simulink model "Block Diagram"  (R2024b)
settings: Solver=VariableStepAuto  StartTime=0.0  StopTime=10.0  RelTol=1e-3
libraries: simulink_extras x43, eeGeneralControl x4
(part 2 of 3)

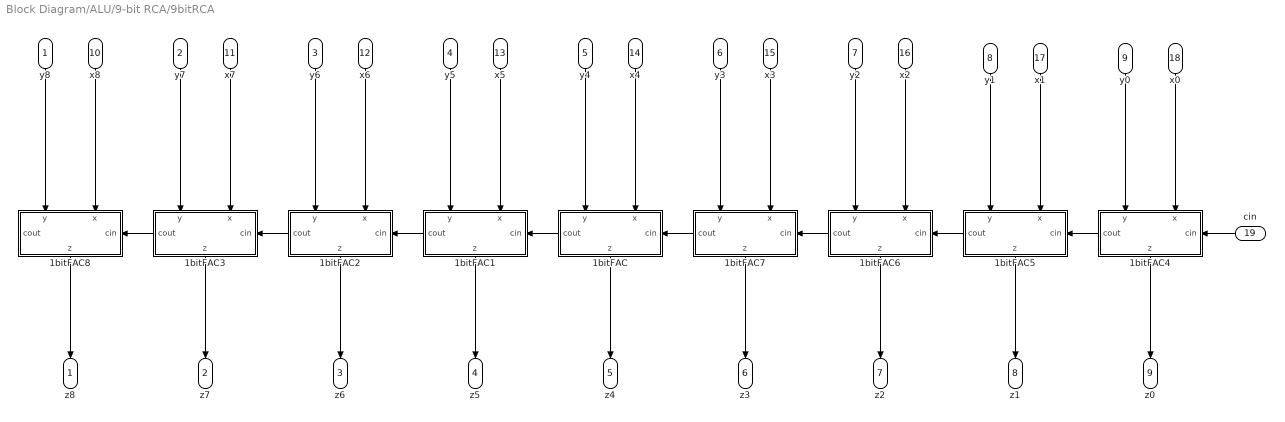
== system Block Diagram/ALU/9-bit RCA/9bitRCA ==
  y8 : Inport
  y7 : Inport  Port=2
  y6 : Inport  Port=3
  y5 : Inport  Port=4
  y4 : Inport  Port=5
  y3 : Inport  Port=6
  y2 : Inport  Port=7
  y1 : Inport  Port=8
  y0 : Inport  Port=9
  x8 : Inport  Port=10
  x7 : Inport  Port=11
  x6 : Inport  Port=12
  x5 : Inport  Port=13
  x4 : Inport  Port=14
  x3 : Inport  Port=15
  x2 : Inport  Port=16
  x1 : Inport  Port=17
  x0 : Inport  Port=18
  cin : Inport  Port=19
  1bitFAC : Subsystem
      settings: PortSchema="{\"entries\":[{\"content\":{\"sides\":[{\"content\":{\"connectorIds\":[\"Out2\"]},\"type\":\"ConnectorPlacement.EquallySpacedRectSide\",\"uuid\":\"3d82b7f9-dc63-4fc7-98b7-23cc47f57a4f\"},{\"content\":{\"connectorIds\":[\"In3\"],\"side\":\"RIGHT\"},\"type\":\"ConnectorPlacement.EquallySpacedRectSide\",\"uuid\":\"46fdb482-606a-4080-9fe4-28ef2e2aeced\"},{\"content\":{\"connectorIds\":[\"In1\",\"In2\"],\"side\":\"TOP\"},\"type\":\"ConnectorPlacement.EquallySpacedRectSide\",\"uuid\":\"27deceb1-bcd8-433c-80a1-5ff3de271941\"},{\"content\":{\"connectorIds\":[\"Out1\"],\"side\":\"BOTTOM\"},\"type\":\"ConnectorPlacement.EquallySpacedRectSide\",\"uuid\":\"1ab1ef58-b8ab-498e-bc4b-e7d01d078e9d\"}]},\"type\":\"ConnectorPlacement.EquallySpacedConnector\",\"uuid\":\"ca739cf1-46eb-41bd-970c-7d220730d652\"}],\"packageUris\":[\"http://schema.mathworks.com/mf0/Connector/R2020b\"],\"version\":\"1.0\"}"
  1bitFAC1 : Subsystem
      settings: PortSchema="{\"entries\":[{\"content\":{\"sides\":[{\"content\":{\"connectorIds\":[\"Out2\"]},\"type\":\"ConnectorPlacement.EquallySpacedRectSide\",\"uuid\":\"3d82b7f9-dc63-4fc7-98b7-23cc47f57a4f\"},{\"content\":{\"connectorIds\":[\"In3\"],\"side\":\"RIGHT\"},\"type\":\"ConnectorPlacement.EquallySpacedRectSide\",\"uuid\":\"46fdb482-606a-4080-9fe4-28ef2e2aeced\"},{\"content\":{\"connectorIds\":[\"In1\",\"In2\"],\"side\":\"TOP\"},\"type\":\"ConnectorPlacement.EquallySpacedRectSide\",\"uuid\":\"27deceb1-bcd8-433c-80a1-5ff3de271941\"},{\"content\":{\"connectorIds\":[\"Out1\"],\"side\":\"BOTTOM\"},\"type\":\"ConnectorPlacement.EquallySpacedRectSide\",\"uuid\":\"1ab1ef58-b8ab-498e-bc4b-e7d01d078e9d\"}]},\"type\":\"ConnectorPlacement.EquallySpacedConnector\",\"uuid\":\"ca739cf1-46eb-41bd-970c-7d220730d652\"}],\"packageUris\":[\"http://schema.mathworks.com/mf0/Connector/R2020b\"],\"version\":\"1.0\"}"
  1bitFAC2 : Subsystem
      settings: PortSchema="{\"entries\":[{\"content\":{\"sides\":[{\"content\":{\"connectorIds\":[\"Out2\"]},\"type\":\"ConnectorPlacement.EquallySpacedRectSide\",\"uuid\":\"3d82b7f9-dc63-4fc7-98b7-23cc47f57a4f\"},{\"content\":{\"connectorIds\":[\"In3\"],\"side\":\"RIGHT\"},\"type\":\"ConnectorPlacement.EquallySpacedRectSide\",\"uuid\":\"46fdb482-606a-4080-9fe4-28ef2e2aeced\"},{\"content\":{\"connectorIds\":[\"In1\",\"In2\"],\"side\":\"TOP\"},\"type\":\"ConnectorPlacement.EquallySpacedRectSide\",\"uuid\":\"27deceb1-bcd8-433c-80a1-5ff3de271941\"},{\"content\":{\"connectorIds\":[\"Out1\"],\"side\":\"BOTTOM\"},\"type\":\"ConnectorPlacement.EquallySpacedRectSide\",\"uuid\":\"1ab1ef58-b8ab-498e-bc4b-e7d01d078e9d\"}]},\"type\":\"ConnectorPlacement.EquallySpacedConnector\",\"uuid\":\"ca739cf1-46eb-41bd-970c-7d220730d652\"}],\"packageUris\":[\"http://schema.mathworks.com/mf0/Connector/R2020b\"],\"version\":\"1.0\"}"
  1bitFAC3 : Subsystem
      settings: PortSchema="{\"entries\":[{\"content\":{\"sides\":[{\"content\":{\"connectorIds\":[\"Out2\"]},\"type\":\"ConnectorPlacement.EquallySpacedRectSide\",\"uuid\":\"3d82b7f9-dc63-4fc7-98b7-23cc47f57a4f\"},{\"content\":{\"connectorIds\":[\"In3\"],\"side\":\"RIGHT\"},\"type\":\"ConnectorPlacement.EquallySpacedRectSide\",\"uuid\":\"46fdb482-606a-4080-9fe4-28ef2e2aeced\"},{\"content\":{\"connectorIds\":[\"In1\",\"In2\"],\"side\":\"TOP\"},\"type\":\"ConnectorPlacement.EquallySpacedRectSide\",\"uuid\":\"27deceb1-bcd8-433c-80a1-5ff3de271941\"},{\"content\":{\"connectorIds\":[\"Out1\"],\"side\":\"BOTTOM\"},\"type\":\"ConnectorPlacement.EquallySpacedRectSide\",\"uuid\":\"1ab1ef58-b8ab-498e-bc4b-e7d01d078e9d\"}]},\"type\":\"ConnectorPlacement.EquallySpacedConnector\",\"uuid\":\"ca739cf1-46eb-41bd-970c-7d220730d652\"}],\"packageUris\":[\"http://schema.mathworks.com/mf0/Connector/R2020b\"],\"version\":\"1.0\"}"
  1bitFAC4 : Subsystem
      settings: PortSchema="{\"entries\":[{\"content\":{\"sides\":[{\"content\":{\"connectorIds\":[\"Out2\"]},\"type\":\"ConnectorPlacement.EquallySpacedRectSide\",\"uuid\":\"3d82b7f9-dc63-4fc7-98b7-23cc47f57a4f\"},{\"content\":{\"connectorIds\":[\"In3\"],\"side\":\"RIGHT\"},\"type\":\"ConnectorPlacement.EquallySpacedRectSide\",\"uuid\":\"46fdb482-606a-4080-9fe4-28ef2e2aeced\"},{\"content\":{\"connectorIds\":[\"In1\",\"In2\"],\"side\":\"TOP\"},\"type\":\"ConnectorPlacement.EquallySpacedRectSide\",\"uuid\":\"27deceb1-bcd8-433c-80a1-5ff3de271941\"},{\"content\":{\"connectorIds\":[\"Out1\"],\"side\":\"BOTTOM\"},\"type\":\"ConnectorPlacement.EquallySpacedRectSide\",\"uuid\":\"1ab1ef58-b8ab-498e-bc4b-e7d01d078e9d\"}]},\"type\":\"ConnectorPlacement.EquallySpacedConnector\",\"uuid\":\"ca739cf1-46eb-41bd-970c-7d220730d652\"}],\"packageUris\":[\"http://schema.mathworks.com/mf0/Connector/R2020b\"],\"version\":\"1.0\"}"
  1bitFAC5 : Subsystem
      settings: PortSchema="{\"entries\":[{\"content\":{\"sides\":[{\"content\":{\"connectorIds\":[\"Out2\"]},\"type\":\"ConnectorPlacement.EquallySpacedRectSide\",\"uuid\":\"3d82b7f9-dc63-4fc7-98b7-23cc47f57a4f\"},{\"content\":{\"connectorIds\":[\"In3\"],\"side\":\"RIGHT\"},\"type\":\"ConnectorPlacement.EquallySpacedRectSide\",\"uuid\":\"46fdb482-606a-4080-9fe4-28ef2e2aeced\"},{\"content\":{\"connectorIds\":[\"In1\",\"In2\"],\"side\":\"TOP\"},\"type\":\"ConnectorPlacement.EquallySpacedRectSide\",\"uuid\":\"27deceb1-bcd8-433c-80a1-5ff3de271941\"},{\"content\":{\"connectorIds\":[\"Out1\"],\"side\":\"BOTTOM\"},\"type\":\"ConnectorPlacement.EquallySpacedRectSide\",\"uuid\":\"1ab1ef58-b8ab-498e-bc4b-e7d01d078e9d\"}]},\"type\":\"ConnectorPlacement.EquallySpacedConnector\",\"uuid\":\"ca739cf1-46eb-41bd-970c-7d220730d652\"}],\"packageUris\":[\"http://schema.mathworks.com/mf0/Connector/R2020b\"],\"version\":\"1.0\"}"
  1bitFAC6 : Subsystem
      settings: PortSchema="{\"entries\":[{\"content\":{\"sides\":[{\"content\":{\"connectorIds\":[\"Out2\"]},\"type\":\"ConnectorPlacement.EquallySpacedRectSide\",\"uuid\":\"3d82b7f9-dc63-4fc7-98b7-23cc47f57a4f\"},{\"content\":{\"connectorIds\":[\"In3\"],\"side\":\"RIGHT\"},\"type\":\"ConnectorPlacement.EquallySpacedRectSide\",\"uuid\":\"46fdb482-606a-4080-9fe4-28ef2e2aeced\"},{\"content\":{\"connectorIds\":[\"In1\",\"In2\"],\"side\":\"TOP\"},\"type\":\"ConnectorPlacement.EquallySpacedRectSide\",\"uuid\":\"27deceb1-bcd8-433c-80a1-5ff3de271941\"},{\"content\":{\"connectorIds\":[\"Out1\"],\"side\":\"BOTTOM\"},\"type\":\"ConnectorPlacement.EquallySpacedRectSide\",\"uuid\":\"1ab1ef58-b8ab-498e-bc4b-e7d01d078e9d\"}]},\"type\":\"ConnectorPlacement.EquallySpacedConnector\",\"uuid\":\"ca739cf1-46eb-41bd-970c-7d220730d652\"}],\"packageUris\":[\"http://schema.mathworks.com/mf0/Connector/R2020b\"],\"version\":\"1.0\"}"
  1bitFAC7 : Subsystem
      settings: PortSchema="{\"entries\":[{\"content\":{\"sides\":[{\"content\":{\"connectorIds\":[\"Out2\"]},\"type\":\"ConnectorPlacement.EquallySpacedRectSide\",\"uuid\":\"3d82b7f9-dc63-4fc7-98b7-23cc47f57a4f\"},{\"content\":{\"connectorIds\":[\"In3\"],\"side\":\"RIGHT\"},\"type\":\"ConnectorPlacement.EquallySpacedRectSide\",\"uuid\":\"46fdb482-606a-4080-9fe4-28ef2e2aeced\"},{\"content\":{\"connectorIds\":[\"In1\",\"In2\"],\"side\":\"TOP\"},\"type\":\"ConnectorPlacement.EquallySpacedRectSide\",\"uuid\":\"27deceb1-bcd8-433c-80a1-5ff3de271941\"},{\"content\":{\"connectorIds\":[\"Out1\"],\"side\":\"BOTTOM\"},\"type\":\"ConnectorPlacement.EquallySpacedRectSide\",\"uuid\":\"1ab1ef58-b8ab-498e-bc4b-e7d01d078e9d\"}]},\"type\":\"ConnectorPlacement.EquallySpacedConnector\",\"uuid\":\"ca739cf1-46eb-41bd-970c-7d220730d652\"}],\"packageUris\":[\"http://schema.mathworks.com/mf0/Connector/R2020b\"],\"version\":\"1.0\"}"
  1bitFAC8 : Subsystem
      settings: PortSchema="{\"entries\":[{\"content\":{\"sides\":[{\"content\":{\"connectorIds\":[\"Out2\"]},\"type\":\"ConnectorPlacement.EquallySpacedRectSide\",\"uuid\":\"3d82b7f9-dc63-4fc7-98b7-23cc47f57a4f\"},{\"content\":{\"connectorIds\":[\"In3\"],\"side\":\"RIGHT\"},\"type\":\"ConnectorPlacement.EquallySpacedRectSide\",\"uuid\":\"46fdb482-606a-4080-9fe4-28ef2e2aeced\"},{\"content\":{\"connectorIds\":[\"In1\",\"In2\"],\"side\":\"TOP\"},\"type\":\"ConnectorPlacement.EquallySpacedRectSide\",\"uuid\":\"27deceb1-bcd8-433c-80a1-5ff3de271941\"},{\"content\":{\"connectorIds\":[\"Out1\"],\"side\":\"BOTTOM\"},\"type\":\"ConnectorPlacement.EquallySpacedRectSide\",\"uuid\":\"1ab1ef58-b8ab-498e-bc4b-e7d01d078e9d\"}]},\"type\":\"ConnectorPlacement.EquallySpacedConnector\",\"uuid\":\"ca739cf1-46eb-41bd-970c-7d220730d652\"}],\"packageUris\":[\"http://schema.mathworks.com/mf0/Connector/R2020b\"],\"version\":\"1.0\"}"
  z8 : Outport
  z7 : Outport  Port=2
  z6 : Outport  Port=3
  z5 : Outport  Port=4
  z4 : Outport  Port=5
  z3 : Outport  Port=6
  z2 : Outport  Port=7
  z1 : Outport  Port=8
  z0 : Outport  Port=9
  wires:
  1bitFAC1/2(cout) -> 1bitFAC2/3(cin)
  1bitFAC5/2(cout) -> 1bitFAC6/3(cin)
  1bitFAC3/2(cout) -> 1bitFAC8/3(cin)
  1bitFAC2/2(cout) -> 1bitFAC3/3(cin)
  1bitFAC/2(cout) -> 1bitFAC1/3(cin)
  1bitFAC7/2(cout) -> 1bitFAC/3(cin)
  1bitFAC6/2(cout) -> 1bitFAC7/3(cin)
  1bitFAC4/2(cout) -> 1bitFAC5/3(cin)
  x0/1 -> 1bitFAC4/2(x)
  x1/1 -> 1bitFAC5/2(x)
  x2/1 -> 1bitFAC6/2(x)
  x3/1 -> 1bitFAC7/2(x)
  x4/1 -> 1bitFAC/2(x)
  x5/1 -> 1bitFAC1/2(x)
  x6/1 -> 1bitFAC2/2(x)
  x7/1 -> 1bitFAC3/2(x)
  x8/1 -> 1bitFAC8/2(x)
  y5/1 -> 1bitFAC1/1(y)
  y7/1 -> 1bitFAC3/1(y)
  y6/1 -> 1bitFAC2/1(y)
  y1/1 -> 1bitFAC5/1(y)
  y4/1 -> 1bitFAC/1(y)
  y2/1 -> 1bitFAC6/1(y)
  y0/1 -> 1bitFAC4/1(y)
  y8/1 -> 1bitFAC8/1(y)
  y3/1 -> 1bitFAC7/1(y)
  1bitFAC4/1(z) -> z0/1
  1bitFAC5/1(z) -> z1/1
  1bitFAC6/1(z) -> z2/1
  1bitFAC7/1(z) -> z3/1
  1bitFAC/1(z) -> z4/1
  1bitFAC1/1(z) -> z5/1
  1bitFAC2/1(z) -> z6/1
  1bitFAC3/1(z) -> z7/1
  1bitFAC8/1(z) -> z8/1
  cin/1 -> 1bitFAC4/3(cin)

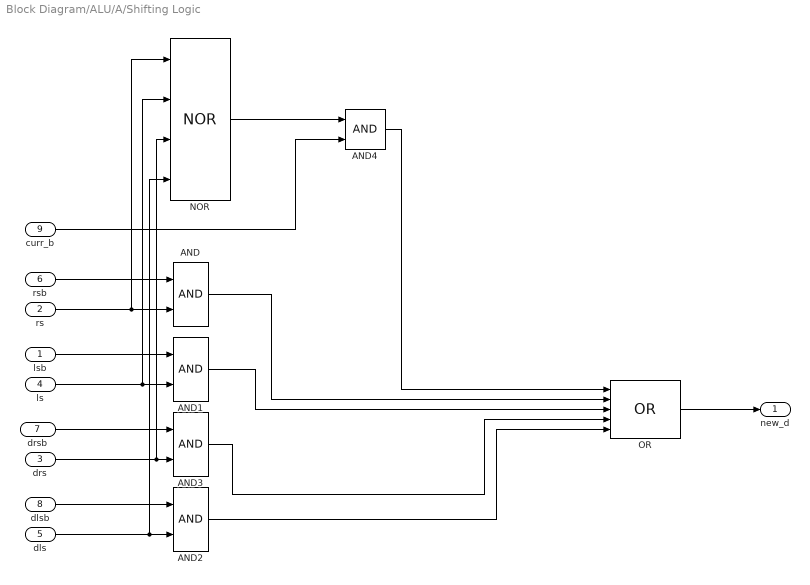
== system Block Diagram/ALU/A/Shifting Logic ==
  lsb : Inport
  rs : Inport  Port=2
  drs : Inport  Port=3
  ls : Inport  Port=4
  dls : Inport  Port=5
  rsb : Inport  Port=6
  drsb : Inport  Port=7
  dlsb : Inport  Port=8
  curr_b : Inport  Port=9
  AND{,1..4} (5 alike) : Logic  IconShape=distinctive  AllPortsSameDT=off  OutDataTypeStr=boolean
  NOR : Logic  Operator=NOR  Inputs=4  IconShape=distinctive  AllPortsSameDT=off  OutDataTypeStr=boolean
  OR : Logic  Operator=OR  Inputs=5  IconShape=distinctive  AllPortsSameDT=off  OutDataTypeStr=boolean
  new_d : Outport
  wires:
  curr_b/1 -> AND4/2
  rsb/1 -> AND/1
  rs/1 -> NOR/1, AND/2
  lsb/1 -> AND1/1
  ls/1 -> NOR/2, AND1/2
  drs/1 -> NOR/3, AND3/2
  drsb/1 -> AND3/1
  dls/1 -> NOR/4, AND2/2
  dlsb/1 -> AND2/1
  NOR/1 -> AND4/1
  AND/1 -> OR/2
  AND1/1 -> OR/3
  AND3/1 -> OR/4
  AND2/1 -> OR/5
  AND4/1 -> OR/1
  OR/1 -> new_d/1

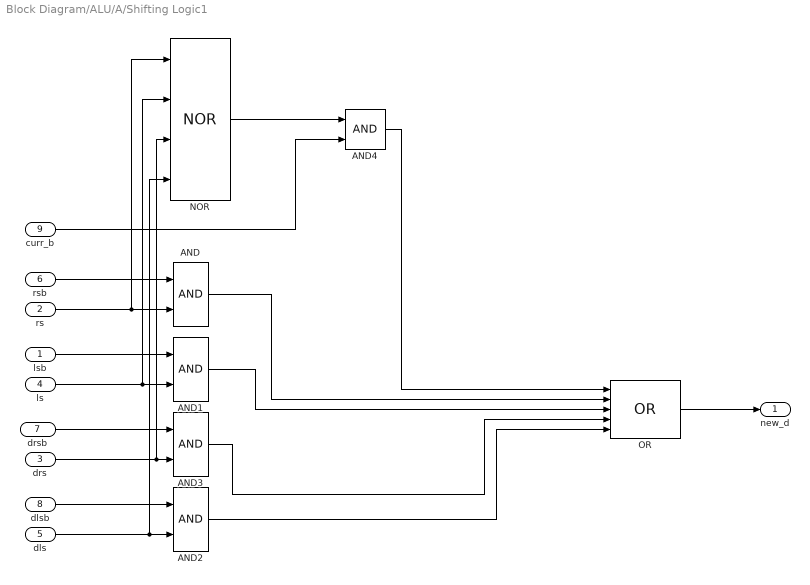
== system Block Diagram/ALU/A/Shifting Logic1 ==
  lsb : Inport
  rs : Inport  Port=2
  drs : Inport  Port=3
  ls : Inport  Port=4
  dls : Inport  Port=5
  rsb : Inport  Port=6
  drsb : Inport  Port=7
  dlsb : Inport  Port=8
  curr_b : Inport  Port=9
  AND{,1..4} (5 alike) : Logic  IconShape=distinctive  AllPortsSameDT=off  OutDataTypeStr=boolean
  NOR : Logic  Operator=NOR  Inputs=4  IconShape=distinctive  AllPortsSameDT=off  OutDataTypeStr=boolean
  OR : Logic  Operator=OR  Inputs=5  IconShape=distinctive  AllPortsSameDT=off  OutDataTypeStr=boolean
  new_d : Outport
  wires:
  curr_b/1 -> AND4/2
  rsb/1 -> AND/1
  rs/1 -> NOR/1, AND/2
  lsb/1 -> AND1/1
  ls/1 -> NOR/2, AND1/2
  drs/1 -> NOR/3, AND3/2
  drsb/1 -> AND3/1
  dls/1 -> NOR/4, AND2/2
  dlsb/1 -> AND2/1
  NOR/1 -> AND4/1
  AND/1 -> OR/2
  AND1/1 -> OR/3
  AND3/1 -> OR/4
  AND2/1 -> OR/5
  AND4/1 -> OR/1
  OR/1 -> new_d/1

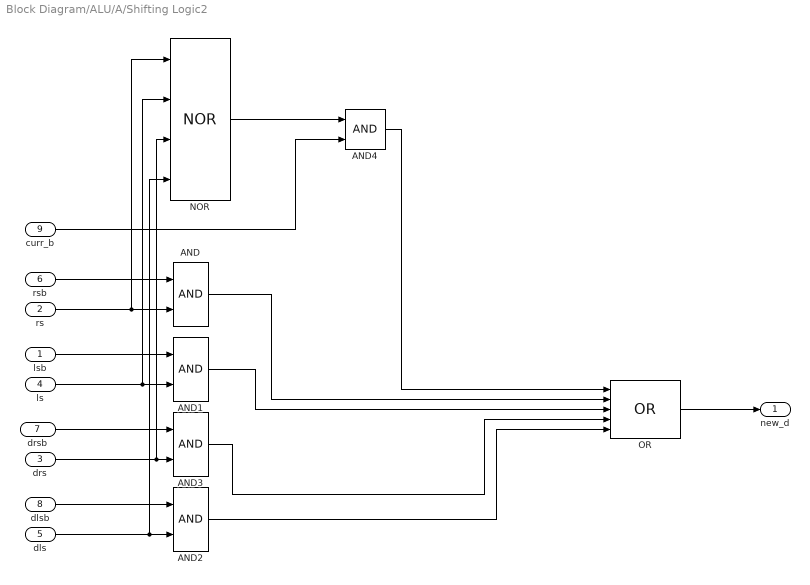
== system Block Diagram/ALU/A/Shifting Logic2 ==
  lsb : Inport
  rs : Inport  Port=2
  drs : Inport  Port=3
  ls : Inport  Port=4
  dls : Inport  Port=5
  rsb : Inport  Port=6
  drsb : Inport  Port=7
  dlsb : Inport  Port=8
  curr_b : Inport  Port=9
  AND{,1..4} (5 alike) : Logic  IconShape=distinctive  AllPortsSameDT=off  OutDataTypeStr=boolean
  NOR : Logic  Operator=NOR  Inputs=4  IconShape=distinctive  AllPortsSameDT=off  OutDataTypeStr=boolean
  OR : Logic  Operator=OR  Inputs=5  IconShape=distinctive  AllPortsSameDT=off  OutDataTypeStr=boolean
  new_d : Outport
  wires:
  curr_b/1 -> AND4/2
  rsb/1 -> AND/1
  rs/1 -> NOR/1, AND/2
  lsb/1 -> AND1/1
  ls/1 -> NOR/2, AND1/2
  drs/1 -> NOR/3, AND3/2
  drsb/1 -> AND3/1
  dls/1 -> NOR/4, AND2/2
  dlsb/1 -> AND2/1
  NOR/1 -> AND4/1
  AND/1 -> OR/2
  AND1/1 -> OR/3
  AND3/1 -> OR/4
  AND2/1 -> OR/5
  AND4/1 -> OR/1
  OR/1 -> new_d/1

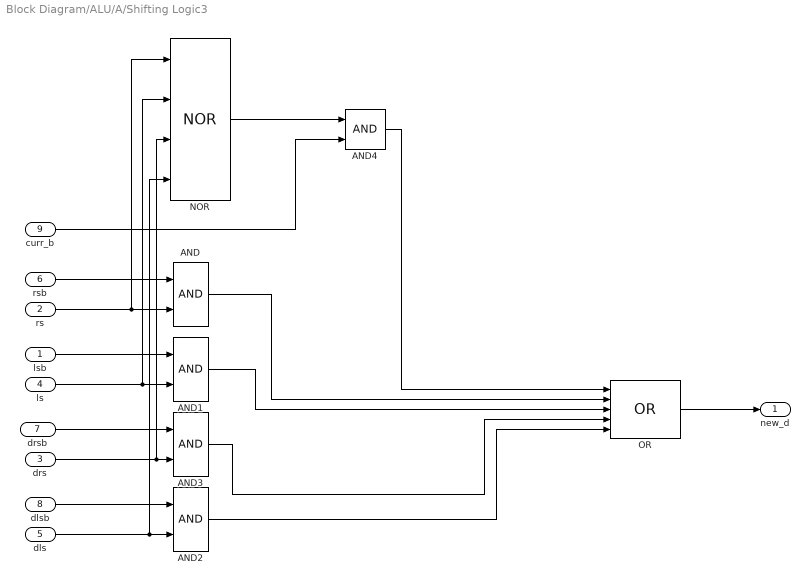
== system Block Diagram/ALU/A/Shifting Logic3 ==
  lsb : Inport
  rs : Inport  Port=2
  drs : Inport  Port=3
  ls : Inport  Port=4
  dls : Inport  Port=5
  rsb : Inport  Port=6
  drsb : Inport  Port=7
  dlsb : Inport  Port=8
  curr_b : Inport  Port=9
  AND{,1..4} (5 alike) : Logic  IconShape=distinctive  AllPortsSameDT=off  OutDataTypeStr=boolean
  NOR : Logic  Operator=NOR  Inputs=4  IconShape=distinctive  AllPortsSameDT=off  OutDataTypeStr=boolean
  OR : Logic  Operator=OR  Inputs=5  IconShape=distinctive  AllPortsSameDT=off  OutDataTypeStr=boolean
  new_d : Outport
  wires:
  curr_b/1 -> AND4/2
  rsb/1 -> AND/1
  rs/1 -> NOR/1, AND/2
  lsb/1 -> AND1/1
  ls/1 -> NOR/2, AND1/2
  drs/1 -> NOR/3, AND3/2
  drsb/1 -> AND3/1
  dls/1 -> NOR/4, AND2/2
  dlsb/1 -> AND2/1
  NOR/1 -> AND4/1
  AND/1 -> OR/2
  AND1/1 -> OR/3
  AND3/1 -> OR/4
  AND2/1 -> OR/5
  AND4/1 -> OR/1
  OR/1 -> new_d/1

== system Block Diagram/ALU/A/Shifting Logic4 ==
  lsb : Inport
  rs : Inport  Port=2
  drs : Inport  Port=3
  ls : Inport  Port=4
  dls : Inport  Port=5
  rsb : Inport  Port=6
  drsb : Inport  Port=7
  dlsb : Inport  Port=8
  curr_b : Inport  Port=9
  AND{,1..4} (5 alike) : Logic  IconShape=distinctive  AllPortsSameDT=off  OutDataTypeStr=boolean
  NOR : Logic  Operator=NOR  Inputs=4  IconShape=distinctive  AllPortsSameDT=off  OutDataTypeStr=boolean
  OR : Logic  Operator=OR  Inputs=5  IconShape=distinctive  AllPortsSameDT=off  OutDataTypeStr=boolean
  new_d : Outport
  wires:
  curr_b/1 -> AND4/2
  rsb/1 -> AND/1
  rs/1 -> NOR/1, AND/2
  lsb/1 -> AND1/1
  ls/1 -> NOR/2, AND1/2
  drs/1 -> NOR/3, AND3/2
  drsb/1 -> AND3/1
  dls/1 -> NOR/4, AND2/2
  dlsb/1 -> AND2/1
  NOR/1 -> AND4/1
  AND/1 -> OR/2
  AND1/1 -> OR/3
  AND3/1 -> OR/4
  AND2/1 -> OR/5
  AND4/1 -> OR/1
  OR/1 -> new_d/1

== system Block Diagram/ALU/A/Shifting Logic5 ==
  lsb : Inport
  rs : Inport  Port=2
  drs : Inport  Port=3
  ls : Inport  Port=4
  dls : Inport  Port=5
  rsb : Inport  Port=6
  drsb : Inport  Port=7
  dlsb : Inport  Port=8
  curr_b : Inport  Port=9
  AND{,1..4} (5 alike) : Logic  IconShape=distinctive  AllPortsSameDT=off  OutDataTypeStr=boolean
  NOR : Logic  Operator=NOR  Inputs=4  IconShape=distinctive  AllPortsSameDT=off  OutDataTypeStr=boolean
  OR : Logic  Operator=OR  Inputs=5  IconShape=distinctive  AllPortsSameDT=off  OutDataTypeStr=boolean
  new_d : Outport
  wires:
  curr_b/1 -> AND4/2
  rsb/1 -> AND/1
  rs/1 -> NOR/1, AND/2
  lsb/1 -> AND1/1
  ls/1 -> NOR/2, AND1/2
  drs/1 -> NOR/3, AND3/2
  drsb/1 -> AND3/1
  dls/1 -> NOR/4, AND2/2
  dlsb/1 -> AND2/1
  NOR/1 -> AND4/1
  AND/1 -> OR/2
  AND1/1 -> OR/3
  AND3/1 -> OR/4
  AND2/1 -> OR/5
  AND4/1 -> OR/1
  OR/1 -> new_d/1

== system Block Diagram/ALU/A/Shifting Logic6 ==
  lsb : Inport
  rs : Inport  Port=2
  drs : Inport  Port=3
  ls : Inport  Port=4
  dls : Inport  Port=5
  rsb : Inport  Port=6
  drsb : Inport  Port=7
  dlsb : Inport  Port=8
  curr_b : Inport  Port=9
  AND{,1..4} (5 alike) : Logic  IconShape=distinctive  AllPortsSameDT=off  OutDataTypeStr=boolean
  NOR : Logic  Operator=NOR  Inputs=4  IconShape=distinctive  AllPortsSameDT=off  OutDataTypeStr=boolean
  OR : Logic  Operator=OR  Inputs=5  IconShape=distinctive  AllPortsSameDT=off  OutDataTypeStr=boolean
  new_d : Outport
  wires:
  curr_b/1 -> AND4/2
  rsb/1 -> AND/1
  rs/1 -> NOR/1, AND/2
  lsb/1 -> AND1/1
  ls/1 -> NOR/2, AND1/2
  drs/1 -> NOR/3, AND3/2
  drsb/1 -> AND3/1
  dls/1 -> NOR/4, AND2/2
  dlsb/1 -> AND2/1
  NOR/1 -> AND4/1
  AND/1 -> OR/2
  AND1/1 -> OR/3
  AND3/1 -> OR/4
  AND2/1 -> OR/5
  AND4/1 -> OR/1
  OR/1 -> new_d/1

== system Block Diagram/ALU/A/Shifting Logic7 ==
  lsb : Inport
  rs : Inport  Port=2
  drs : Inport  Port=3
  ls : Inport  Port=4
  dls : Inport  Port=5
  rsb : Inport  Port=6
  drsb : Inport  Port=7
  dlsb : Inport  Port=8
  curr_b : Inport  Port=9
  AND{,1..4} (5 alike) : Logic  IconShape=distinctive  AllPortsSameDT=off  OutDataTypeStr=boolean
  NOR : Logic  Operator=NOR  Inputs=4  IconShape=distinctive  AllPortsSameDT=off  OutDataTypeStr=boolean
  OR : Logic  Operator=OR  Inputs=5  IconShape=distinctive  AllPortsSameDT=off  OutDataTypeStr=boolean
  new_d : Outport
  wires:
  curr_b/1 -> AND4/2
  rsb/1 -> AND/1
  rs/1 -> NOR/1, AND/2
  lsb/1 -> AND1/1
  ls/1 -> NOR/2, AND1/2
  drs/1 -> NOR/3, AND3/2
  drsb/1 -> AND3/1
  dls/1 -> NOR/4, AND2/2
  dlsb/1 -> AND2/1
  NOR/1 -> AND4/1
  AND/1 -> OR/2
  AND1/1 -> OR/3
  AND3/1 -> OR/4
  AND2/1 -> OR/5
  AND4/1 -> OR/1
  OR/1 -> new_d/1

== system Block Diagram/ALU/A/Tristate Selector ==
  In1 : Inport
  Action Port : ActionPort
  Out1 : Outport
  wires:
  In1/1 -> Out1/1

== system Block Diagram/ALU/A/Tristate Selector1 ==
  In1 : Inport
  Action Port : ActionPort
  Out1 : Outport
  wires:
  In1/1 -> Out1/1

== system Block Diagram/ALU/A/Tristate Selector2 ==
  In1 : Inport
  Action Port : ActionPort
  Out1 : Outport
  wires:
  In1/1 -> Out1/1

== system Block Diagram/ALU/A/Tristate Selector3 ==
  In1 : Inport
  Action Port : ActionPort
  Out1 : Outport
  wires:
  In1/1 -> Out1/1

== system Block Diagram/ALU/A/Tristate Selector4 ==
  In1 : Inport
  Action Port : ActionPort
  Out1 : Outport
  wires:
  In1/1 -> Out1/1

== system Block Diagram/ALU/A/Tristate Selector5 ==
  In1 : Inport
  Action Port : ActionPort
  Out1 : Outport
  wires:
  In1/1 -> Out1/1

== system Block Diagram/ALU/A/Tristate Selector6 ==
  In1 : Inport
  Action Port : ActionPort
  Out1 : Outport
  wires:
  In1/1 -> Out1/1

== system Block Diagram/ALU/A/Tristate Selector7 ==
  In1 : Inport
  Action Port : ActionPort
  Out1 : Outport
  wires:
  In1/1 -> Out1/1

== system Block Diagram/ALU/B/Shifting Logic ==
  lsb : Inport
  rs : Inport  Port=2
  drs : Inport  Port=3
  ls : Inport  Port=4
  dls : Inport  Port=5
  rsb : Inport  Port=6
  drsb : Inport  Port=7
  dlsb : Inport  Port=8
  curr_b : Inport  Port=9
  AND{,1..4} (5 alike) : Logic  IconShape=distinctive  AllPortsSameDT=off  OutDataTypeStr=boolean
  NOR : Logic  Operator=NOR  Inputs=4  IconShape=distinctive  AllPortsSameDT=off  OutDataTypeStr=boolean
  OR : Logic  Operator=OR  Inputs=5  IconShape=distinctive  AllPortsSameDT=off  OutDataTypeStr=boolean
  new_d : Outport
  wires:
  curr_b/1 -> AND4/2
  rsb/1 -> AND/1
  rs/1 -> NOR/1, AND/2
  lsb/1 -> AND1/1
  ls/1 -> NOR/2, AND1/2
  drs/1 -> NOR/3, AND3/2
  drsb/1 -> AND3/1
  dls/1 -> NOR/4, AND2/2
  dlsb/1 -> AND2/1
  NOR/1 -> AND4/1
  AND/1 -> OR/2
  AND1/1 -> OR/3
  AND3/1 -> OR/4
  AND2/1 -> OR/5
  AND4/1 -> OR/1
  OR/1 -> new_d/1

== system Block Diagram/ALU/B/Shifting Logic1 ==
  lsb : Inport
  rs : Inport  Port=2
  drs : Inport  Port=3
  ls : Inport  Port=4
  dls : Inport  Port=5
  rsb : Inport  Port=6
  drsb : Inport  Port=7
  dlsb : Inport  Port=8
  curr_b : Inport  Port=9
  AND{,1..4} (5 alike) : Logic  IconShape=distinctive  AllPortsSameDT=off  OutDataTypeStr=boolean
  NOR : Logic  Operator=NOR  Inputs=4  IconShape=distinctive  AllPortsSameDT=off  OutDataTypeStr=boolean
  OR : Logic  Operator=OR  Inputs=5  IconShape=distinctive  AllPortsSameDT=off  OutDataTypeStr=boolean
  new_d : Outport
  wires:
  curr_b/1 -> AND4/2
  rsb/1 -> AND/1
  rs/1 -> NOR/1, AND/2
  lsb/1 -> AND1/1
  ls/1 -> NOR/2, AND1/2
  drs/1 -> NOR/3, AND3/2
  drsb/1 -> AND3/1
  dls/1 -> NOR/4, AND2/2
  dlsb/1 -> AND2/1
  NOR/1 -> AND4/1
  AND/1 -> OR/2
  AND1/1 -> OR/3
  AND3/1 -> OR/4
  AND2/1 -> OR/5
  AND4/1 -> OR/1
  OR/1 -> new_d/1

== system Block Diagram/ALU/B/Shifting Logic2 ==
  lsb : Inport
  rs : Inport  Port=2
  drs : Inport  Port=3
  ls : Inport  Port=4
  dls : Inport  Port=5
  rsb : Inport  Port=6
  drsb : Inport  Port=7
  dlsb : Inport  Port=8
  curr_b : Inport  Port=9
  AND{,1..4} (5 alike) : Logic  IconShape=distinctive  AllPortsSameDT=off  OutDataTypeStr=boolean
  NOR : Logic  Operator=NOR  Inputs=4  IconShape=distinctive  AllPortsSameDT=off  OutDataTypeStr=boolean
  OR : Logic  Operator=OR  Inputs=5  IconShape=distinctive  AllPortsSameDT=off  OutDataTypeStr=boolean
  new_d : Outport
  wires:
  curr_b/1 -> AND4/2
  rsb/1 -> AND/1
  rs/1 -> NOR/1, AND/2
  lsb/1 -> AND1/1
  ls/1 -> NOR/2, AND1/2
  drs/1 -> NOR/3, AND3/2
  drsb/1 -> AND3/1
  dls/1 -> NOR/4, AND2/2
  dlsb/1 -> AND2/1
  NOR/1 -> AND4/1
  AND/1 -> OR/2
  AND1/1 -> OR/3
  AND3/1 -> OR/4
  AND2/1 -> OR/5
  AND4/1 -> OR/1
  OR/1 -> new_d/1

== system Block Diagram/ALU/B/Shifting Logic3 ==
  lsb : Inport
  rs : Inport  Port=2
  drs : Inport  Port=3
  ls : Inport  Port=4
  dls : Inport  Port=5
  rsb : Inport  Port=6
  drsb : Inport  Port=7
  dlsb : Inport  Port=8
  curr_b : Inport  Port=9
  AND{,1..4} (5 alike) : Logic  IconShape=distinctive  AllPortsSameDT=off  OutDataTypeStr=boolean
  NOR : Logic  Operator=NOR  Inputs=4  IconShape=distinctive  AllPortsSameDT=off  OutDataTypeStr=boolean
  OR : Logic  Operator=OR  Inputs=5  IconShape=distinctive  AllPortsSameDT=off  OutDataTypeStr=boolean
  new_d : Outport
  wires:
  curr_b/1 -> AND4/2
  rsb/1 -> AND/1
  rs/1 -> NOR/1, AND/2
  lsb/1 -> AND1/1
  ls/1 -> NOR/2, AND1/2
  drs/1 -> NOR/3, AND3/2
  drsb/1 -> AND3/1
  dls/1 -> NOR/4, AND2/2
  dlsb/1 -> AND2/1
  NOR/1 -> AND4/1
  AND/1 -> OR/2
  AND1/1 -> OR/3
  AND3/1 -> OR/4
  AND2/1 -> OR/5
  AND4/1 -> OR/1
  OR/1 -> new_d/1

== system Block Diagram/ALU/B/Shifting Logic4 ==
  lsb : Inport
  rs : Inport  Port=2
  drs : Inport  Port=3
  ls : Inport  Port=4
  dls : Inport  Port=5
  rsb : Inport  Port=6
  drsb : Inport  Port=7
  dlsb : Inport  Port=8
  curr_b : Inport  Port=9
  AND{,1..4} (5 alike) : Logic  IconShape=distinctive  AllPortsSameDT=off  OutDataTypeStr=boolean
  NOR : Logic  Operator=NOR  Inputs=4  IconShape=distinctive  AllPortsSameDT=off  OutDataTypeStr=boolean
  OR : Logic  Operator=OR  Inputs=5  IconShape=distinctive  AllPortsSameDT=off  OutDataTypeStr=boolean
  new_d : Outport
  wires:
  curr_b/1 -> AND4/2
  rsb/1 -> AND/1
  rs/1 -> NOR/1, AND/2
  lsb/1 -> AND1/1
  ls/1 -> NOR/2, AND1/2
  drs/1 -> NOR/3, AND3/2
  drsb/1 -> AND3/1
  dls/1 -> NOR/4, AND2/2
  dlsb/1 -> AND2/1
  NOR/1 -> AND4/1
  AND/1 -> OR/2
  AND1/1 -> OR/3
  AND3/1 -> OR/4
  AND2/1 -> OR/5
  AND4/1 -> OR/1
  OR/1 -> new_d/1

== system Block Diagram/ALU/B/Shifting Logic5 ==
  lsb : Inport
  rs : Inport  Port=2
  drs : Inport  Port=3
  ls : Inport  Port=4
  dls : Inport  Port=5
  rsb : Inport  Port=6
  drsb : Inport  Port=7
  dlsb : Inport  Port=8
  curr_b : Inport  Port=9
  AND{,1..4} (5 alike) : Logic  IconShape=distinctive  AllPortsSameDT=off  OutDataTypeStr=boolean
  NOR : Logic  Operator=NOR  Inputs=4  IconShape=distinctive  AllPortsSameDT=off  OutDataTypeStr=boolean
  OR : Logic  Operator=OR  Inputs=5  IconShape=distinctive  AllPortsSameDT=off  OutDataTypeStr=boolean
  new_d : Outport
  wires:
  curr_b/1 -> AND4/2
  rsb/1 -> AND/1
  rs/1 -> NOR/1, AND/2
  lsb/1 -> AND1/1
  ls/1 -> NOR/2, AND1/2
  drs/1 -> NOR/3, AND3/2
  drsb/1 -> AND3/1
  dls/1 -> NOR/4, AND2/2
  dlsb/1 -> AND2/1
  NOR/1 -> AND4/1
  AND/1 -> OR/2
  AND1/1 -> OR/3
  AND3/1 -> OR/4
  AND2/1 -> OR/5
  AND4/1 -> OR/1
  OR/1 -> new_d/1

== system Block Diagram/ALU/B/Shifting Logic6 ==
  lsb : Inport
  rs : Inport  Port=2
  drs : Inport  Port=3
  ls : Inport  Port=4
  dls : Inport  Port=5
  rsb : Inport  Port=6
  drsb : Inport  Port=7
  dlsb : Inport  Port=8
  curr_b : Inport  Port=9
  AND{,1..4} (5 alike) : Logic  IconShape=distinctive  AllPortsSameDT=off  OutDataTypeStr=boolean
  NOR : Logic  Operator=NOR  Inputs=4  IconShape=distinctive  AllPortsSameDT=off  OutDataTypeStr=boolean
  OR : Logic  Operator=OR  Inputs=5  IconShape=distinctive  AllPortsSameDT=off  OutDataTypeStr=boolean
  new_d : Outport
  wires:
  curr_b/1 -> AND4/2
  rsb/1 -> AND/1
  rs/1 -> NOR/1, AND/2
  lsb/1 -> AND1/1
  ls/1 -> NOR/2, AND1/2
  drs/1 -> NOR/3, AND3/2
  drsb/1 -> AND3/1
  dls/1 -> NOR/4, AND2/2
  dlsb/1 -> AND2/1
  NOR/1 -> AND4/1
  AND/1 -> OR/2
  AND1/1 -> OR/3
  AND3/1 -> OR/4
  AND2/1 -> OR/5
  AND4/1 -> OR/1
  OR/1 -> new_d/1

== system Block Diagram/ALU/B/Shifting Logic7 ==
  lsb : Inport
  rs : Inport  Port=2
  drs : Inport  Port=3
  ls : Inport  Port=4
  dls : Inport  Port=5
  rsb : Inport  Port=6
  drsb : Inport  Port=7
  dlsb : Inport  Port=8
  curr_b : Inport  Port=9
  AND{,1..4} (5 alike) : Logic  IconShape=distinctive  AllPortsSameDT=off  OutDataTypeStr=boolean
  NOR : Logic  Operator=NOR  Inputs=4  IconShape=distinctive  AllPortsSameDT=off  OutDataTypeStr=boolean
  OR : Logic  Operator=OR  Inputs=5  IconShape=distinctive  AllPortsSameDT=off  OutDataTypeStr=boolean
  new_d : Outport
  wires:
  curr_b/1 -> AND4/2
  rsb/1 -> AND/1
  rs/1 -> NOR/1, AND/2
  lsb/1 -> AND1/1
  ls/1 -> NOR/2, AND1/2
  drs/1 -> NOR/3, AND3/2
  drsb/1 -> AND3/1
  dls/1 -> NOR/4, AND2/2
  dlsb/1 -> AND2/1
  NOR/1 -> AND4/1
  AND/1 -> OR/2
  AND1/1 -> OR/3
  AND3/1 -> OR/4
  AND2/1 -> OR/5
  AND4/1 -> OR/1
  OR/1 -> new_d/1

== system Block Diagram/ALU/B/Tristate Selector ==
  In1 : Inport
  Action Port : ActionPort
  Out1 : Outport
  wires:
  In1/1 -> Out1/1

== system Block Diagram/ALU/B/Tristate Selector1 ==
  In1 : Inport
  Action Port : ActionPort
  Out1 : Outport
  wires:
  In1/1 -> Out1/1

== system Block Diagram/ALU/B/Tristate Selector2 ==
  In1 : Inport
  Action Port : ActionPort
  Out1 : Outport
  wires:
  In1/1 -> Out1/1

== system Block Diagram/ALU/B/Tristate Selector3 ==
  In1 : Inport
  Action Port : ActionPort
  Out1 : Outport
  wires:
  In1/1 -> Out1/1

== system Block Diagram/ALU/B/Tristate Selector4 ==
  In1 : Inport
  Action Port : ActionPort
  Out1 : Outport
  wires:
  In1/1 -> Out1/1

== system Block Diagram/ALU/B/Tristate Selector5 ==
  In1 : Inport
  Action Port : ActionPort
  Out1 : Outport
  wires:
  In1/1 -> Out1/1

== system Block Diagram/ALU/B/Tristate Selector6 ==
  In1 : Inport
  Action Port : ActionPort
  Out1 : Outport
  wires:
  In1/1 -> Out1/1

== system Block Diagram/ALU/B/Tristate Selector7 ==
  In1 : Inport
  Action Port : ActionPort
  Out1 : Outport
  wires:
  In1/1 -> Out1/1

== system Block Diagram/ALU/Control Unit/modulo-3 phase counter ==
  begin : Inport
  end : Inport  Port=2
  rst : Inport  Port=3
  clk : Inport  Port=4
  2-3 decoder : Subsystem
      settings: PortSchema="{\"entries\":[{\"content\":{\"sides\":[{\"content\":{},\"type\":\"ConnectorPlacement.EquallySpacedRectSide\",\"uuid\":\"d16f9b83-c968-4926-93cb-d3adbbf76b75\"},{\"content\":{\"side\":\"RIGHT\"},\"type\":\"ConnectorPlacement.EquallySpacedRectSide\",\"uuid\":\"0a52a34b-f708-4e43-b48b-8fd019c86006\"},{\"content\":{\"connectorIds\":[\"In1\",\"In2\"],\"side\":\"TOP\"},\"type\":\"ConnectorPlacement.EquallySpacedRectSide\",\"uuid\":\"f648a8d6-b46a-4076-94ce-f281b5d51bf9\"},{\"content\":{\"connectorIds\":[\"Out1\",\"Out2\",\"Out3\",\"Out4\"],\"side\":\"BOTTOM\"},\"type\":\"ConnectorPlacement.EquallySpacedRectSide\",\"uuid\":\"ba6aebfe-4d74-4323-b62f-c75d8d5cf386\"}]},\"type\":\"ConnectorPlacement.EquallySpacedConnector\",\"uuid\":\"329b5702-50d6-4aa0-9bd3-18c943ae0e62\"}],\"packageUris\":[\"http://schema.mathworks.com/mf0/Connector/R2020b\"],\"version\":\"1.0\"}"
  AND : Logic  IconShape=distinctive  AllPortsSameDT=off  OutDataTypeStr=boolean
  OR : Logic  Operator=OR  IconShape=distinctive  AllPortsSameDT=off  OutDataTypeStr=boolean
  Set-Reset Flip-Flop : eeGeneralControl/Set-Reset Flip-Flop  LabelModeActiveChoice=Discrete  UndefState=Set  Q0=0  Ts=-1
      settings: LibrarySourceBlock=ee_sl_lib/General Control/Set-Reset Flip-Flop
  modulo-3 counter : Subsystem
      settings: PortSchema="{\"entries\":[{\"content\":{\"sides\":[{\"content\":{\"connectorIds\":[\"In1\",\"In2\"]},\"type\":\"ConnectorPlacement.EquallySpacedRectSide\",\"uuid\":\"495221cc-c37a-49fe-a40a-f2d85f7abf45\"},{\"content\":{\"side\":\"RIGHT\"},\"type\":\"ConnectorPlacement.EquallySpacedRectSide\",\"uuid\":\"b157812d-780c-4ff2-a3b6-c41211f61e25\"},{\"content\":{\"side\":\"TOP\"},\"type\":\"ConnectorPlacement.EquallySpacedRectSide\",\"uuid\":\"49483137-7145-40d7-9abf-b1a953ad9dc1\"},{\"content\":{\"connectorIds\":[\"Out1\",\"Out2\"],\"side\":\"BOTTOM\"},\"type\":\"ConnectorPlacement.EquallySpacedRectSide\",\"uuid\":\"09f8707d-71f2-4e33-ac3d-267e76ed2b64\"}]},\"type\":\"ConnectorPlacement.EquallySpacedConnector\",\"uuid\":\"85b6cdfb-ddce-400c-92bb-856bec3d38f0\"}],\"packageUris\":[\"http://schema.mathworks.com/mf0/Connector/R2020b\"],\"version\":\"1.0\"}"
  Ph4 : Outport
  Ph3 : Outport  Port=2
  Ph2 : Outport  Port=3
  Ph1 : Outport  Port=4
  wires:
  2-3 decoder/2(Ph2) -> Ph3/1
  modulo-3 counter/2(b0) -> 2-3 decoder/2(d0)
  2-3 decoder/4(Ph0) -> Ph1/1
  modulo-3 counter/1(b1) -> 2-3 decoder/1(d1)
  clk/1 -> AND/1
  2-3 decoder/3(Ph1) -> Ph2/1
  begin/1 -> Set-Reset Flip-Flop/1
  end/1 -> OR/1, Set-Reset Flip-Flop/2
  AND/1 -> modulo-3 counter/1(clk)
  Set-Reset Flip-Flop/1 -> AND/2
  rst/1 -> OR/2
  OR/1 -> modulo-3 counter/2(rst)
  2-3 decoder/1(Ph3) -> Ph4/1

== system Block Diagram/ALU/Q/Shifting Logic ==
  lsb : Inport
  rs : Inport  Port=2
  drs : Inport  Port=3
  ls : Inport  Port=4
  dls : Inport  Port=5
  rsb : Inport  Port=6
  drsb : Inport  Port=7
  dlsb : Inport  Port=8
  curr_b : Inport  Port=9
  AND{,1..4} (5 alike) : Logic  IconShape=distinctive  AllPortsSameDT=off  OutDataTypeStr=boolean
  NOR : Logic  Operator=NOR  Inputs=4  IconShape=distinctive  AllPortsSameDT=off  OutDataTypeStr=boolean
  OR : Logic  Operator=OR  Inputs=5  IconShape=distinctive  AllPortsSameDT=off  OutDataTypeStr=boolean
  new_d : Outport
  wires:
  curr_b/1 -> AND4/2
  rsb/1 -> AND/1
  rs/1 -> NOR/1, AND/2
  lsb/1 -> AND1/1
  ls/1 -> NOR/2, AND1/2
  drs/1 -> NOR/3, AND3/2
  drsb/1 -> AND3/1
  dls/1 -> NOR/4, AND2/2
  dlsb/1 -> AND2/1
  NOR/1 -> AND4/1
  AND/1 -> OR/2
  AND1/1 -> OR/3
  AND3/1 -> OR/4
  AND2/1 -> OR/5
  AND4/1 -> OR/1
  OR/1 -> new_d/1

== system Block Diagram/ALU/Q/Shifting Logic1 ==
  lsb : Inport
  rs : Inport  Port=2
  drs : Inport  Port=3
  ls : Inport  Port=4
  dls : Inport  Port=5
  rsb : Inport  Port=6
  drsb : Inport  Port=7
  dlsb : Inport  Port=8
  curr_b : Inport  Port=9
  AND{,1..4} (5 alike) : Logic  IconShape=distinctive  AllPortsSameDT=off  OutDataTypeStr=boolean
  NOR : Logic  Operator=NOR  Inputs=4  IconShape=distinctive  AllPortsSameDT=off  OutDataTypeStr=boolean
  OR : Logic  Operator=OR  Inputs=5  IconShape=distinctive  AllPortsSameDT=off  OutDataTypeStr=boolean
  new_d : Outport
  wires:
  curr_b/1 -> AND4/2
  rsb/1 -> AND/1
  rs/1 -> NOR/1, AND/2
  lsb/1 -> AND1/1
  ls/1 -> NOR/2, AND1/2
  drs/1 -> NOR/3, AND3/2
  drsb/1 -> AND3/1
  dls/1 -> NOR/4, AND2/2
  dlsb/1 -> AND2/1
  NOR/1 -> AND4/1
  AND/1 -> OR/2
  AND1/1 -> OR/3
  AND3/1 -> OR/4
  AND2/1 -> OR/5
  AND4/1 -> OR/1
  OR/1 -> new_d/1

== system Block Diagram/ALU/Q/Shifting Logic2 ==
  lsb : Inport
  rs : Inport  Port=2
  drs : Inport  Port=3
  ls : Inport  Port=4
  dls : Inport  Port=5
  rsb : Inport  Port=6
  drsb : Inport  Port=7
  dlsb : Inport  Port=8
  curr_b : Inport  Port=9
  AND{,1..4} (5 alike) : Logic  IconShape=distinctive  AllPortsSameDT=off  OutDataTypeStr=boolean
  NOR : Logic  Operator=NOR  Inputs=4  IconShape=distinctive  AllPortsSameDT=off  OutDataTypeStr=boolean
  OR : Logic  Operator=OR  Inputs=5  IconShape=distinctive  AllPortsSameDT=off  OutDataTypeStr=boolean
  new_d : Outport
  wires:
  curr_b/1 -> AND4/2
  rsb/1 -> AND/1
  rs/1 -> NOR/1, AND/2
  lsb/1 -> AND1/1
  ls/1 -> NOR/2, AND1/2
  drs/1 -> NOR/3, AND3/2
  drsb/1 -> AND3/1
  dls/1 -> NOR/4, AND2/2
  dlsb/1 -> AND2/1
  NOR/1 -> AND4/1
  AND/1 -> OR/2
  AND1/1 -> OR/3
  AND3/1 -> OR/4
  AND2/1 -> OR/5
  AND4/1 -> OR/1
  OR/1 -> new_d/1

== system Block Diagram/ALU/Q/Shifting Logic3 ==
  lsb : Inport
  rs : Inport  Port=2
  drs : Inport  Port=3
  ls : Inport  Port=4
  dls : Inport  Port=5
  rsb : Inport  Port=6
  drsb : Inport  Port=7
  dlsb : Inport  Port=8
  curr_b : Inport  Port=9
  AND{,1..4} (5 alike) : Logic  IconShape=distinctive  AllPortsSameDT=off  OutDataTypeStr=boolean
  NOR : Logic  Operator=NOR  Inputs=4  IconShape=distinctive  AllPortsSameDT=off  OutDataTypeStr=boolean
  OR : Logic  Operator=OR  Inputs=5  IconShape=distinctive  AllPortsSameDT=off  OutDataTypeStr=boolean
  new_d : Outport
  wires:
  curr_b/1 -> AND4/2
  rsb/1 -> AND/1
  rs/1 -> NOR/1, AND/2
  lsb/1 -> AND1/1
  ls/1 -> NOR/2, AND1/2
  drs/1 -> NOR/3, AND3/2
  drsb/1 -> AND3/1
  dls/1 -> NOR/4, AND2/2
  dlsb/1 -> AND2/1
  NOR/1 -> AND4/1
  AND/1 -> OR/2
  AND1/1 -> OR/3
  AND3/1 -> OR/4
  AND2/1 -> OR/5
  AND4/1 -> OR/1
  OR/1 -> new_d/1

== system Block Diagram/ALU/Q/Shifting Logic4 ==
  lsb : Inport
  rs : Inport  Port=2
  drs : Inport  Port=3
  ls : Inport  Port=4
  dls : Inport  Port=5
  rsb : Inport  Port=6
  drsb : Inport  Port=7
  dlsb : Inport  Port=8
  curr_b : Inport  Port=9
  AND{,1..4} (5 alike) : Logic  IconShape=distinctive  AllPortsSameDT=off  OutDataTypeStr=boolean
  NOR : Logic  Operator=NOR  Inputs=4  IconShape=distinctive  AllPortsSameDT=off  OutDataTypeStr=boolean
  OR : Logic  Operator=OR  Inputs=5  IconShape=distinctive  AllPortsSameDT=off  OutDataTypeStr=boolean
  new_d : Outport
  wires:
  curr_b/1 -> AND4/2
  rsb/1 -> AND/1
  rs/1 -> NOR/1, AND/2
  lsb/1 -> AND1/1
  ls/1 -> NOR/2, AND1/2
  drs/1 -> NOR/3, AND3/2
  drsb/1 -> AND3/1
  dls/1 -> NOR/4, AND2/2
  dlsb/1 -> AND2/1
  NOR/1 -> AND4/1
  AND/1 -> OR/2
  AND1/1 -> OR/3
  AND3/1 -> OR/4
  AND2/1 -> OR/5
  AND4/1 -> OR/1
  OR/1 -> new_d/1

== system Block Diagram/ALU/Q/Shifting Logic5 ==
  lsb : Inport
  rs : Inport  Port=2
  drs : Inport  Port=3
  ls : Inport  Port=4
  dls : Inport  Port=5
  rsb : Inport  Port=6
  drsb : Inport  Port=7
  dlsb : Inport  Port=8
  curr_b : Inport  Port=9
  AND{,1..4} (5 alike) : Logic  IconShape=distinctive  AllPortsSameDT=off  OutDataTypeStr=boolean
  NOR : Logic  Operator=NOR  Inputs=4  IconShape=distinctive  AllPortsSameDT=off  OutDataTypeStr=boolean
  OR : Logic  Operator=OR  Inputs=5  IconShape=distinctive  AllPortsSameDT=off  OutDataTypeStr=boolean
  new_d : Outport
  wires:
  curr_b/1 -> AND4/2
  rsb/1 -> AND/1
  rs/1 -> NOR/1, AND/2
  lsb/1 -> AND1/1
  ls/1 -> NOR/2, AND1/2
  drs/1 -> NOR/3, AND3/2
  drsb/1 -> AND3/1
  dls/1 -> NOR/4, AND2/2
  dlsb/1 -> AND2/1
  NOR/1 -> AND4/1
  AND/1 -> OR/2
  AND1/1 -> OR/3
  AND3/1 -> OR/4
  AND2/1 -> OR/5
  AND4/1 -> OR/1
  OR/1 -> new_d/1

== system Block Diagram/ALU/Q/Shifting Logic6 ==
  lsb : Inport
  rs : Inport  Port=2
  drs : Inport  Port=3
  ls : Inport  Port=4
  dls : Inport  Port=5
  rsb : Inport  Port=6
  drsb : Inport  Port=7
  dlsb : Inport  Port=8
  curr_b : Inport  Port=9
  AND{,1..4} (5 alike) : Logic  IconShape=distinctive  AllPortsSameDT=off  OutDataTypeStr=boolean
  NOR : Logic  Operator=NOR  Inputs=4  IconShape=distinctive  AllPortsSameDT=off  OutDataTypeStr=boolean
  OR : Logic  Operator=OR  Inputs=5  IconShape=distinctive  AllPortsSameDT=off  OutDataTypeStr=boolean
  new_d : Outport
  wires:
  curr_b/1 -> AND4/2
  rsb/1 -> AND/1
  rs/1 -> NOR/1, AND/2
  lsb/1 -> AND1/1
  ls/1 -> NOR/2, AND1/2
  drs/1 -> NOR/3, AND3/2
  drsb/1 -> AND3/1
  dls/1 -> NOR/4, AND2/2
  dlsb/1 -> AND2/1
  NOR/1 -> AND4/1
  AND/1 -> OR/2
  AND1/1 -> OR/3
  AND3/1 -> OR/4
  AND2/1 -> OR/5
  AND4/1 -> OR/1
  OR/1 -> new_d/1

== system Block Diagram/ALU/Q/Shifting Logic7 ==
  lsb : Inport
  rs : Inport  Port=2
  drs : Inport  Port=3
  ls : Inport  Port=4
  dls : Inport  Port=5
  rsb : Inport  Port=6
  drsb : Inport  Port=7
  dlsb : Inport  Port=8
  curr_b : Inport  Port=9
  AND{,1..4} (5 alike) : Logic  IconShape=distinctive  AllPortsSameDT=off  OutDataTypeStr=boolean
  NOR : Logic  Operator=NOR  Inputs=4  IconShape=distinctive  AllPortsSameDT=off  OutDataTypeStr=boolean
  OR : Logic  Operator=OR  Inputs=5  IconShape=distinctive  AllPortsSameDT=off  OutDataTypeStr=boolean
  new_d : Outport
  wires:
  curr_b/1 -> AND4/2
  rsb/1 -> AND/1
  rs/1 -> NOR/1, AND/2
  lsb/1 -> AND1/1
  ls/1 -> NOR/2, AND1/2
  drs/1 -> NOR/3, AND3/2
  drsb/1 -> AND3/1
  dls/1 -> NOR/4, AND2/2
  dlsb/1 -> AND2/1
  NOR/1 -> AND4/1
  AND/1 -> OR/2
  AND1/1 -> OR/3
  AND3/1 -> OR/4
  AND2/1 -> OR/5
  AND4/1 -> OR/1
  OR/1 -> new_d/1

== system Block Diagram/ALU/Q/Tristate Selector ==
  In1 : Inport
  Action Port : ActionPort
  Out1 : Outport
  wires:
  In1/1 -> Out1/1

== system Block Diagram/ALU/Q/Tristate Selector1 ==
  In1 : Inport
  Action Port : ActionPort
  Out1 : Outport
  wires:
  In1/1 -> Out1/1

== system Block Diagram/ALU/Q/Tristate Selector2 ==
  In1 : Inport
  Action Port : ActionPort
  Out1 : Outport
  wires:
  In1/1 -> Out1/1

== system Block Diagram/ALU/Q/Tristate Selector3 ==
  In1 : Inport
  Action Port : ActionPort
  Out1 : Outport
  wires:
  In1/1 -> Out1/1

== system Block Diagram/ALU/Q/Tristate Selector4 ==
  In1 : Inport
  Action Port : ActionPort
  Out1 : Outport
  wires:
  In1/1 -> Out1/1

== system Block Diagram/ALU/Q/Tristate Selector5 ==
  In1 : Inport
  Action Port : ActionPort
  Out1 : Outport
  wires:
  In1/1 -> Out1/1

== system Block Diagram/ALU/Q/Tristate Selector6 ==
  In1 : Inport
  Action Port : ActionPort
  Out1 : Outport
  wires:
  In1/1 -> Out1/1

== system Block Diagram/ALU/Q/Tristate Selector7 ==
  In1 : Inport
  Action Port : ActionPort
  Out1 : Outport
  wires:
  In1/1 -> Out1/1

== system Block Diagram/ALU/Q'/Shifting Logic ==
  lsb : Inport
  rs : Inport  Port=2
  drs : Inport  Port=3
  ls : Inport  Port=4
  dls : Inport  Port=5
  rsb : Inport  Port=6
  drsb : Inport  Port=7
  dlsb : Inport  Port=8
  curr_b : Inport  Port=9
  AND{,1..4} (5 alike) : Logic  IconShape=distinctive  AllPortsSameDT=off  OutDataTypeStr=boolean
  NOR : Logic  Operator=NOR  Inputs=4  IconShape=distinctive  AllPortsSameDT=off  OutDataTypeStr=boolean
  OR : Logic  Operator=OR  Inputs=5  IconShape=distinctive  AllPortsSameDT=off  OutDataTypeStr=boolean
  new_d : Outport
  wires:
  curr_b/1 -> AND4/2
  rsb/1 -> AND/1
  rs/1 -> NOR/1, AND/2
  lsb/1 -> AND1/1
  ls/1 -> NOR/2, AND1/2
  drs/1 -> NOR/3, AND3/2
  drsb/1 -> AND3/1
  dls/1 -> NOR/4, AND2/2
  dlsb/1 -> AND2/1
  NOR/1 -> AND4/1
  AND/1 -> OR/2
  AND1/1 -> OR/3
  AND3/1 -> OR/4
  AND2/1 -> OR/5
  AND4/1 -> OR/1
  OR/1 -> new_d/1

== system Block Diagram/ALU/Q'/Shifting Logic1 ==
  lsb : Inport
  rs : Inport  Port=2
  drs : Inport  Port=3
  ls : Inport  Port=4
  dls : Inport  Port=5
  rsb : Inport  Port=6
  drsb : Inport  Port=7
  dlsb : Inport  Port=8
  curr_b : Inport  Port=9
  AND{,1..4} (5 alike) : Logic  IconShape=distinctive  AllPortsSameDT=off  OutDataTypeStr=boolean
  NOR : Logic  Operator=NOR  Inputs=4  IconShape=distinctive  AllPortsSameDT=off  OutDataTypeStr=boolean
  OR : Logic  Operator=OR  Inputs=5  IconShape=distinctive  AllPortsSameDT=off  OutDataTypeStr=boolean
  new_d : Outport
  wires:
  curr_b/1 -> AND4/2
  rsb/1 -> AND/1
  rs/1 -> NOR/1, AND/2
  lsb/1 -> AND1/1
  ls/1 -> NOR/2, AND1/2
  drs/1 -> NOR/3, AND3/2
  drsb/1 -> AND3/1
  dls/1 -> NOR/4, AND2/2
  dlsb/1 -> AND2/1
  NOR/1 -> AND4/1
  AND/1 -> OR/2
  AND1/1 -> OR/3
  AND3/1 -> OR/4
  AND2/1 -> OR/5
  AND4/1 -> OR/1
  OR/1 -> new_d/1

== system Block Diagram/ALU/Q'/Shifting Logic2 ==
  lsb : Inport
  rs : Inport  Port=2
  drs : Inport  Port=3
  ls : Inport  Port=4
  dls : Inport  Port=5
  rsb : Inport  Port=6
  drsb : Inport  Port=7
  dlsb : Inport  Port=8
  curr_b : Inport  Port=9
  AND{,1..4} (5 alike) : Logic  IconShape=distinctive  AllPortsSameDT=off  OutDataTypeStr=boolean
  NOR : Logic  Operator=NOR  Inputs=4  IconShape=distinctive  AllPortsSameDT=off  OutDataTypeStr=boolean
  OR : Logic  Operator=OR  Inputs=5  IconShape=distinctive  AllPortsSameDT=off  OutDataTypeStr=boolean
  new_d : Outport
  wires:
  curr_b/1 -> AND4/2
  rsb/1 -> AND/1
  rs/1 -> NOR/1, AND/2
  lsb/1 -> AND1/1
  ls/1 -> NOR/2, AND1/2
  drs/1 -> NOR/3, AND3/2
  drsb/1 -> AND3/1
  dls/1 -> NOR/4, AND2/2
  dlsb/1 -> AND2/1
  NOR/1 -> AND4/1
  AND/1 -> OR/2
  AND1/1 -> OR/3
  AND3/1 -> OR/4
  AND2/1 -> OR/5
  AND4/1 -> OR/1
  OR/1 -> new_d/1

== system Block Diagram/ALU/Q'/Shifting Logic3 ==
  lsb : Inport
  rs : Inport  Port=2
  drs : Inport  Port=3
  ls : Inport  Port=4
  dls : Inport  Port=5
  rsb : Inport  Port=6
  drsb : Inport  Port=7
  dlsb : Inport  Port=8
  curr_b : Inport  Port=9
  AND{,1..4} (5 alike) : Logic  IconShape=distinctive  AllPortsSameDT=off  OutDataTypeStr=boolean
  NOR : Logic  Operator=NOR  Inputs=4  IconShape=distinctive  AllPortsSameDT=off  OutDataTypeStr=boolean
  OR : Logic  Operator=OR  Inputs=5  IconShape=distinctive  AllPortsSameDT=off  OutDataTypeStr=boolean
  new_d : Outport
  wires:
  curr_b/1 -> AND4/2
  rsb/1 -> AND/1
  rs/1 -> NOR/1, AND/2
  lsb/1 -> AND1/1
  ls/1 -> NOR/2, AND1/2
  drs/1 -> NOR/3, AND3/2
  drsb/1 -> AND3/1
  dls/1 -> NOR/4, AND2/2
  dlsb/1 -> AND2/1
  NOR/1 -> AND4/1
  AND/1 -> OR/2
  AND1/1 -> OR/3
  AND3/1 -> OR/4
  AND2/1 -> OR/5
  AND4/1 -> OR/1
  OR/1 -> new_d/1

== system Block Diagram/ALU/Q'/Shifting Logic4 ==
  lsb : Inport
  rs : Inport  Port=2
  drs : Inport  Port=3
  ls : Inport  Port=4
  dls : Inport  Port=5
  rsb : Inport  Port=6
  drsb : Inport  Port=7
  dlsb : Inport  Port=8
  curr_b : Inport  Port=9
  AND{,1..4} (5 alike) : Logic  IconShape=distinctive  AllPortsSameDT=off  OutDataTypeStr=boolean
  NOR : Logic  Operator=NOR  Inputs=4  IconShape=distinctive  AllPortsSameDT=off  OutDataTypeStr=boolean
  OR : Logic  Operator=OR  Inputs=5  IconShape=distinctive  AllPortsSameDT=off  OutDataTypeStr=boolean
  new_d : Outport
  wires:
  curr_b/1 -> AND4/2
  rsb/1 -> AND/1
  rs/1 -> NOR/1, AND/2
  lsb/1 -> AND1/1
  ls/1 -> NOR/2, AND1/2
  drs/1 -> NOR/3, AND3/2
  drsb/1 -> AND3/1
  dls/1 -> NOR/4, AND2/2
  dlsb/1 -> AND2/1
  NOR/1 -> AND4/1
  AND/1 -> OR/2
  AND1/1 -> OR/3
  AND3/1 -> OR/4
  AND2/1 -> OR/5
  AND4/1 -> OR/1
  OR/1 -> new_d/1

== system Block Diagram/ALU/Q'/Shifting Logic5 ==
  lsb : Inport
  rs : Inport  Port=2
  drs : Inport  Port=3
  ls : Inport  Port=4
  dls : Inport  Port=5
  rsb : Inport  Port=6
  drsb : Inport  Port=7
  dlsb : Inport  Port=8
  curr_b : Inport  Port=9
  AND{,1..4} (5 alike) : Logic  IconShape=distinctive  AllPortsSameDT=off  OutDataTypeStr=boolean
  NOR : Logic  Operator=NOR  Inputs=4  IconShape=distinctive  AllPortsSameDT=off  OutDataTypeStr=boolean
  OR : Logic  Operator=OR  Inputs=5  IconShape=distinctive  AllPortsSameDT=off  OutDataTypeStr=boolean
  new_d : Outport
  wires:
  curr_b/1 -> AND4/2
  rsb/1 -> AND/1
  rs/1 -> NOR/1, AND/2
  lsb/1 -> AND1/1
  ls/1 -> NOR/2, AND1/2
  drs/1 -> NOR/3, AND3/2
  drsb/1 -> AND3/1
  dls/1 -> NOR/4, AND2/2
  dlsb/1 -> AND2/1
  NOR/1 -> AND4/1
  AND/1 -> OR/2
  AND1/1 -> OR/3
  AND3/1 -> OR/4
  AND2/1 -> OR/5
  AND4/1 -> OR/1
  OR/1 -> new_d/1

== system Block Diagram/ALU/Q'/Shifting Logic6 ==
  lsb : Inport
  rs : Inport  Port=2
  drs : Inport  Port=3
  ls : Inport  Port=4
  dls : Inport  Port=5
  rsb : Inport  Port=6
  drsb : Inport  Port=7
  dlsb : Inport  Port=8
  curr_b : Inport  Port=9
  AND{,1..4} (5 alike) : Logic  IconShape=distinctive  AllPortsSameDT=off  OutDataTypeStr=boolean
  NOR : Logic  Operator=NOR  Inputs=4  IconShape=distinctive  AllPortsSameDT=off  OutDataTypeStr=boolean
  OR : Logic  Operator=OR  Inputs=5  IconShape=distinctive  AllPortsSameDT=off  OutDataTypeStr=boolean
  new_d : Outport
  wires:
  curr_b/1 -> AND4/2
  rsb/1 -> AND/1
  rs/1 -> NOR/1, AND/2
  lsb/1 -> AND1/1
  ls/1 -> NOR/2, AND1/2
  drs/1 -> NOR/3, AND3/2
  drsb/1 -> AND3/1
  dls/1 -> NOR/4, AND2/2
  dlsb/1 -> AND2/1
  NOR/1 -> AND4/1
  AND/1 -> OR/2
  AND1/1 -> OR/3
  AND3/1 -> OR/4
  AND2/1 -> OR/5
  AND4/1 -> OR/1
  OR/1 -> new_d/1

== system Block Diagram/ALU/Q'/Shifting Logic7 ==
  lsb : Inport
  rs : Inport  Port=2
  drs : Inport  Port=3
  ls : Inport  Port=4
  dls : Inport  Port=5
  rsb : Inport  Port=6
  drsb : Inport  Port=7
  dlsb : Inport  Port=8
  curr_b : Inport  Port=9
  AND{,1..4} (5 alike) : Logic  IconShape=distinctive  AllPortsSameDT=off  OutDataTypeStr=boolean
  NOR : Logic  Operator=NOR  Inputs=4  IconShape=distinctive  AllPortsSameDT=off  OutDataTypeStr=boolean
  OR : Logic  Operator=OR  Inputs=5  IconShape=distinctive  AllPortsSameDT=off  OutDataTypeStr=boolean
  new_d : Outport
  wires:
  curr_b/1 -> AND4/2
  rsb/1 -> AND/1
  rs/1 -> NOR/1, AND/2
  lsb/1 -> AND1/1
  ls/1 -> NOR/2, AND1/2
  drs/1 -> NOR/3, AND3/2
  drsb/1 -> AND3/1
  dls/1 -> NOR/4, AND2/2
  dlsb/1 -> AND2/1
  NOR/1 -> AND4/1
  AND/1 -> OR/2
  AND1/1 -> OR/3
  AND3/1 -> OR/4
  AND2/1 -> OR/5
  AND4/1 -> OR/1
  OR/1 -> new_d/1

== system Block Diagram/ALU/Q'/Tristate Selector ==
  In1 : Inport
  Action Port : ActionPort
  Out1 : Outport
  wires:
  In1/1 -> Out1/1

== system Block Diagram/ALU/Q'/Tristate Selector1 ==
  In1 : Inport
  Action Port : ActionPort
  Out1 : Outport
  wires:
  In1/1 -> Out1/1

== system Block Diagram/ALU/Q'/Tristate Selector2 ==
  In1 : Inport
  Action Port : ActionPort
  Out1 : Outport
  wires:
  In1/1 -> Out1/1

== system Block Diagram/ALU/Q'/Tristate Selector3 ==
  In1 : Inport
  Action Port : ActionPort
  Out1 : Outport
  wires:
  In1/1 -> Out1/1

== system Block Diagram/ALU/Q'/Tristate Selector4 ==
  In1 : Inport
  Action Port : ActionPort
  Out1 : Outport
  wires:
  In1/1 -> Out1/1

== system Block Diagram/ALU/Q'/Tristate Selector5 ==
  In1 : Inport
  Action Port : ActionPort
  Out1 : Outport
  wires:
  In1/1 -> Out1/1

== system Block Diagram/ALU/Q'/Tristate Selector6 ==
  In1 : Inport
  Action Port : ActionPort
  Out1 : Outport
  wires:
  In1/1 -> Out1/1

== system Block Diagram/ALU/Q'/Tristate Selector7 ==
  In1 : Inport
  Action Port : ActionPort
  Out1 : Outport
  wires:
  In1/1 -> Out1/1

== system Block Diagram/ALU/cnt1/3-bit counter ==
  clk : Inport
  rst : Inport  Port=2
  D Flip-Flop : simulink_extras/Flip Flops/D Flip-Flop
  D Flip-Flop1 : simulink_extras/Flip Flops/D Flip-Flop
  D Flip-Flop2 : simulink_extras/Flip Flops/D Flip-Flop
  NOT : Logic  Operator=NOT  IconShape=distinctive  AllPortsSameDT=off  OutDataTypeStr=boolean
  b0 : Outport
  b1 : Outport  Port=2
  b2 : Outport  Port=3
  wires:
  rst/1 -> NOT/1
  D Flip-Flop/2 -> b0/1, D Flip-Flop/1, D Flip-Flop1/2
  D Flip-Flop1/2 -> D Flip-Flop2/2, b1/1, D Flip-Flop1/1
  NOT/1 -> D Flip-Flop/3, D Flip-Flop2/3, D Flip-Flop1/3
  clk/1 -> D Flip-Flop/2
  D Flip-Flop2/2 -> b2/1, D Flip-Flop2/1

== system Block Diagram/ALU/cnt2/3-bit counter ==
  clk : Inport
  rst : Inport  Port=2
  D Flip-Flop : simulink_extras/Flip Flops/D Flip-Flop
  D Flip-Flop1 : simulink_extras/Flip Flops/D Flip-Flop
  D Flip-Flop2 : simulink_extras/Flip Flops/D Flip-Flop
  NOT : Logic  Operator=NOT  IconShape=distinctive  AllPortsSameDT=off  OutDataTypeStr=boolean
  b0 : Outport
  b1 : Outport  Port=2
  b2 : Outport  Port=3
  wires:
  rst/1 -> NOT/1
  D Flip-Flop/2 -> b0/1, D Flip-Flop/1, D Flip-Flop1/2
  D Flip-Flop1/2 -> D Flip-Flop2/2, b1/1, D Flip-Flop1/1
  NOT/1 -> D Flip-Flop/3, D Flip-Flop2/3, D Flip-Flop1/3
  clk/1 -> D Flip-Flop/2
  D Flip-Flop2/2 -> b2/1, D Flip-Flop2/1

== system Block Diagram/ALU/cnt2/3-bit counter1 ==
  rst : Inport
  clk : Inport  Port=2
  D Flip-Flop : simulink_extras/Flip Flops/D Flip-Flop
  D Flip-Flop1 : simulink_extras/Flip Flops/D Flip-Flop
  D Flip-Flop2 : simulink_extras/Flip Flops/D Flip-Flop
  NOT : Logic  Operator=NOT  IconShape=distinctive  AllPortsSameDT=off  OutDataTypeStr=boolean
  b0 : Outport
  b1 : Outport  Port=2
  b2 : Outport  Port=3
  wires:
  rst/1 -> NOT/1
  D Flip-Flop/2 -> b0/1, D Flip-Flop/1, D Flip-Flop1/2
  D Flip-Flop1/2 -> D Flip-Flop2/2, b1/1, D Flip-Flop1/1
  NOT/1 -> D Flip-Flop/3, D Flip-Flop2/3, D Flip-Flop1/3
  clk/1 -> D Flip-Flop/2
  D Flip-Flop2/2 -> b2/1, D Flip-Flop2/1

== system Block Diagram/ALU/9-bit RCA/9bitRCA/1bitFAC ==
  y : Inport
  x : Inport  Port=2
  cin : Inport  Port=3
  AND : Logic  IconShape=distinctive  AllPortsSameDT=off  OutDataTypeStr=boolean
  AND1 : Logic  IconShape=distinctive  AllPortsSameDT=off  OutDataTypeStr=boolean
  AND2 : Logic  IconShape=distinctive  AllPortsSameDT=off  OutDataTypeStr=boolean
  OR : Logic  Operator=OR  Inputs=3  IconShape=distinctive  AllPortsSameDT=off  OutDataTypeStr=boolean
  XOR : Logic  Operator=XOR  Inputs=3  IconShape=distinctive  AllPortsSameDT=off  OutDataTypeStr=boolean
  z : Outport
  cout : Outport  Port=2
  wires:
  y/1 -> AND2/1, AND/2, XOR/2
  x/1 -> AND1/1, AND/1, XOR/1
  cin/1 -> AND2/2, AND1/2, XOR/3
  XOR/1 -> z/1
  OR/1 -> cout/1
  AND/1 -> OR/1
  AND1/1 -> OR/2
  AND2/1 -> OR/3

== system Block Diagram/ALU/9-bit RCA/9bitRCA/1bitFAC1 ==
  y : Inport
  x : Inport  Port=2
  cin : Inport  Port=3
  AND : Logic  IconShape=distinctive  AllPortsSameDT=off  OutDataTypeStr=boolean
  AND1 : Logic  IconShape=distinctive  AllPortsSameDT=off  OutDataTypeStr=boolean
  AND2 : Logic  IconShape=distinctive  AllPortsSameDT=off  OutDataTypeStr=boolean
  OR : Logic  Operator=OR  Inputs=3  IconShape=distinctive  AllPortsSameDT=off  OutDataTypeStr=boolean
  XOR : Logic  Operator=XOR  Inputs=3  IconShape=distinctive  AllPortsSameDT=off  OutDataTypeStr=boolean
  z : Outport
  cout : Outport  Port=2
  wires:
  y/1 -> AND2/1, AND/2, XOR/2
  x/1 -> AND1/1, AND/1, XOR/1
  cin/1 -> AND2/2, AND1/2, XOR/3
  XOR/1 -> z/1
  OR/1 -> cout/1
  AND/1 -> OR/1
  AND1/1 -> OR/2
  AND2/1 -> OR/3
